simulink model "LAB5A"  (R2020a)
settings: Solver=ode45  StartTime=0.0  StopTime=0.05  RelTol=1e-6  EnableMultiTasking=on
values from neighbouring files (symbols this model uses):
  f = 25    [LAB2.m]
  Ls = 0.087    [LAB2.m]
  Rs = 0.5    [LAB2.m]
  uftopp = 325    [LAB2.m]
settings Model: Creator=ielolof  LastModifiedBy=98all
settings DataIOCC: LimitDataPoints=on  SaveFormat=Array  SignalLoggingSaveFormat=ModelDataLogs  ReturnWorkspaceOutputs=off  SignalLoggingName=sigsOut
settings OptimizationCC: ExpressionDepthLimit=2147483647  InitFltsAndDblsToZero=on  LifeSpan=inf
settings DebuggingCC: SaveWithParameterizedLinksMsg=none  UnderspecifiedInitializationDetection=Classic  MergeDetectMultiDrivingBlocksExec=none  SignalResolutionControl=TryResolveAllWithWarning  MultiTaskDSMMsg=warning  MultiTaskCondExecSysMsg=none  FcnCallInpInsideContextMsg=warning  StateNameClashWarn=warning  SFUnexpectedBacktrackingDiag=warning  SFNoUnconditionalDefaultTransitionDiag=warning  SFExecutionAtInitializationDiag=none  ArithmeticOperatorsInVariantConditions=warning
settings HardwareCC: ProdBitPerPointer=32  ProdBitPerSizeT=32  ProdBitPerPtrDiffT=32  ProdLargestAtomicFloat=None  ProdIntDivRoundTo=Undefined  ProdEndianess=Unspecified  ProdWordSize=32  ProdHWDeviceType=32-bit Generic  TargetUnknown=on
settings ModelReferenceCC: PropagateSignalLabelsOutOfModel=off
settings SFSimCC: SimUseLocalCustomCode=off  CustomCodeUndefinedFunction=UseInterfaceOnly
settings RTWCC: RTWUseLocalCustomCode=off
settings CodeAppCC: StateflowObjectComments=on
settings GRTTargetCC: TargetLangStandard=C89/C90 (ANSI)  ModelReferenceCompliant=off  CompOptLevelCompliant=off  CombineOutputUpdateFcns=off  MatFileLogging=off  GRTInterface=on
settings ConfigComp: CovMetricSettings=dw  CovHtmlReporting=on  CovSaveCumulativeToWorkspaceVar=on  CovSaveSingleToWorkspaceVar=on  CovExternalEMLEnable=off  CovSFcnEnable=off

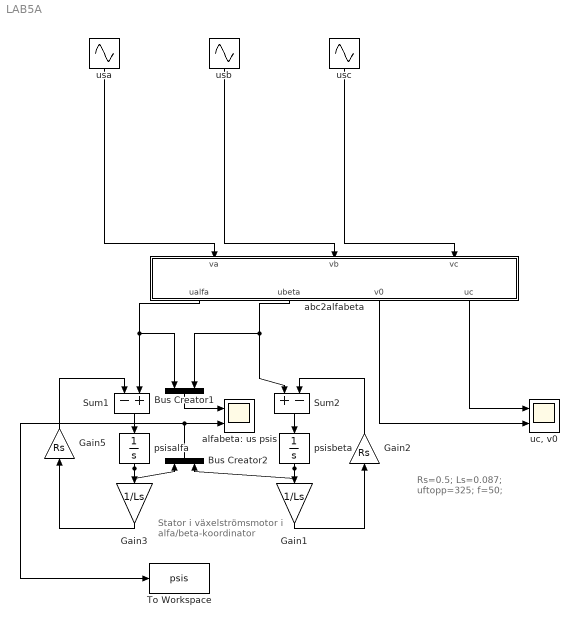
== system LAB5A ==
  note: Rs=0.5;
      | Ls=0.087;
      | uftopp=325;
      | f=50;
  note: Stator i växelströmsmotor
      | i alfa/beta-koordinator
  Bus Creator1 : BusCreator  Inputs=2
  Bus Creator2 : BusCreator  Inputs=2
  Gain1 : Gain  Gain=1/Ls  SaturateOnIntegerOverflow=on  OutDataTypeStr=Inherit: Same as input  ParamDataTypeStr=Inherit: Same as input
  Gain2 : Gain  Gain=Rs  SaturateOnIntegerOverflow=on  OutDataTypeStr=Inherit: Same as input  ParamDataTypeStr=Inherit: Same as input
  Gain3 : Gain  Gain=1/Ls  SaturateOnIntegerOverflow=on  OutDataTypeStr=Inherit: Same as input  ParamDataTypeStr=Inherit: Same as input
  Gain5 : Gain  Gain=Rs  SaturateOnIntegerOverflow=on  OutDataTypeStr=Inherit: Same as input  ParamDataTypeStr=Inherit: Same as input
  Sum1 : Sum  Inputs=-+  SaturateOnIntegerOverflow=on
  Sum2 : Sum  Inputs=+-  SaturateOnIntegerOverflow=on
  To Workspace : ToWorkspace  VariableName=psis  SampleTime=-1
  abc2alfabeta : Subsystem
  alfabeta: us psis : Scope  NumInputPorts=2
  psisalfa : Integrator  InitialCondition=-1.24
  psisbeta : Integrator
  "uc, v0" : Scope  NumInputPorts=2
  usa : Sin  Amplitude=uftopp  Frequency=2*pi*f  SampleTime=0
  usb : Sin  Amplitude=uftopp  Frequency=2*pi*f  Phase=-2*pi/3  SampleTime=0
  usc : Sin  Amplitude=uftopp  Frequency=2*pi*f  Phase=-4*pi/3  SampleTime=0
  wires:
  Sum1/1 -> psisalfa/1
  psisalfa/1 -> Gain3/1, Bus Creator2/1
  Gain3/1 -> Gain5/1
  Gain5/1 -> Sum1/1
  usa/1 -> abc2alfabeta/1(va)
  usb/1 -> abc2alfabeta/2(vb)
  usc/1 -> abc2alfabeta/3(vc)
  abc2alfabeta/1(ualfa) -> Sum1/2, Bus Creator1/1
  Sum2/1 -> psisbeta/1
  psisbeta/1 -> Gain1/1, Bus Creator2/2
  Gain1/1 -> Gain2/1
  Gain2/1 -> Sum2/2
  abc2alfabeta/2(ubeta) -> Sum2/1, Bus Creator1/2
  Bus Creator1/1 -> alfabeta: us psis/1
  Bus Creator2/1 -> alfabeta: us psis/2, To Workspace/1
  abc2alfabeta/3(v0) -> "uc, v0"/2
  abc2alfabeta/4(uc) -> "uc, v0"/1

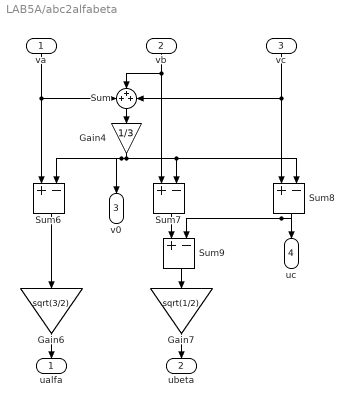
== system LAB5A/abc2alfabeta ==
  va : Inport
  vb : Inport  Port=2
  vc : Inport  Port=3
  Gain4 : Gain  Gain=1/3  SaturateOnIntegerOverflow=on  OutDataTypeStr=Inherit: Same as input  ParamDataTypeStr=Inherit: Same as input
  Gain6 : Gain  Gain=sqrt(3/2)  SaturateOnIntegerOverflow=on  OutDataTypeStr=Inherit: Same as input  ParamDataTypeStr=Inherit: Same as input
  Gain7 : Gain  Gain=sqrt(1/2)  SaturateOnIntegerOverflow=on  OutDataTypeStr=Inherit: Same as input  ParamDataTypeStr=Inherit: Same as input
  Sum : Sum  Inputs=+++
  Sum{6..9} (4 alike) : Sum  Inputs=+-  InputSameDT=on  SaturateOnIntegerOverflow=on  OutDataTypeStr=Inherit: Same as first input
  ualfa : Outport  VectorParamsAs1DForOutWhenUnconnected=off
  ubeta : Outport  Port=2  VectorParamsAs1DForOutWhenUnconnected=off
  v0 : Outport  Port=3  VectorParamsAs1DForOutWhenUnconnected=off
  uc : Outport  Port=4  VectorParamsAs1DForOutWhenUnconnected=off
  wires:
  va/1 -> Sum6/1, Sum/1
  vc/1 -> Sum8/1, Sum/3
  vb/1 -> Sum7/1, Sum/2
  Sum/1 -> Gain4/1
  Gain4/1 -> Sum7/2, Sum8/2, Sum6/2, v0/1
  Sum6/1 -> Gain6/1
  Sum9/1 -> Gain7/1
  Sum7/1 -> Sum9/1
  Sum8/1 -> Sum9/2, uc/1
  Gain6/1 -> ualfa/1
  Gain7/1 -> ubeta/1
